simulink model "capitol6prob1"  (R2013a)
settings: Solver=ode45  StartTime=0.0  StopTime=200  RelTol=1e-3
undefined symbols (not defined in the file): des, gcbh
settings Model: Creator=user  LastModifiedBy=user

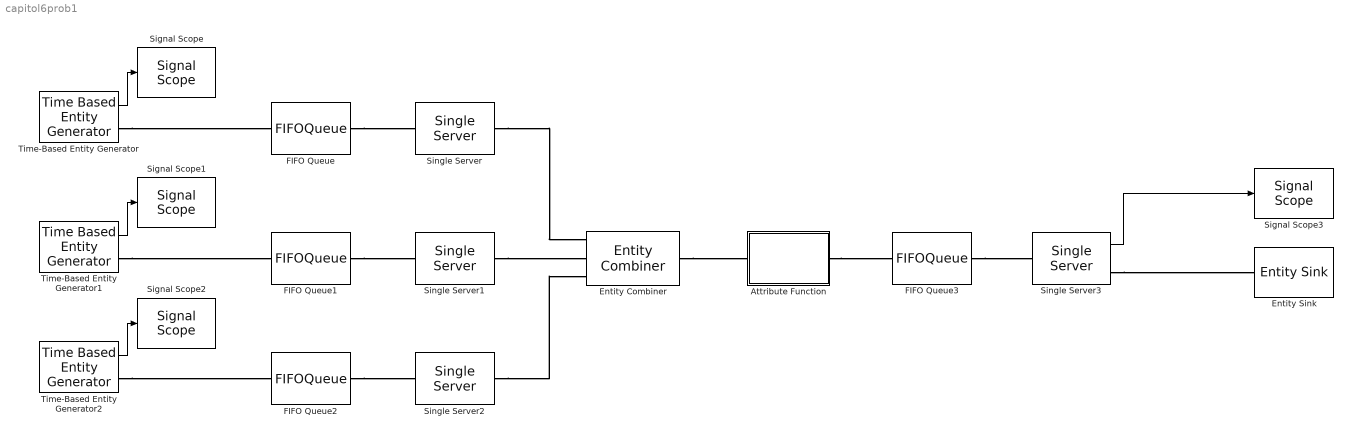
== system capitol6prob1 ==
  Attribute Function : Subsystem  LoadFcn=des.afb.attributefunction_support(gcb,'LoadFcn');  StartFcn=des.afb.attributefunction_support(gcb,'StartFcn');  mask(Attribute Function){OutputNamePrefix=out_}
      mask prompts: OutputNamePrefix "Prefix name"
      settings: CopyFcn=des.afb.attributefunction_support(gcb,'CopyFcn');  OpenFcn=des.afb.attributefunction_support(gcb,'OpenFcn');  ErrorFcn=des.afb.error_redirect
      mask Help: slhelp(gcbh)
      mask Display: image(des_iconLoad('attribFunction.jpg'),'center');
  Entity Combiner : EntityCombiner
  Entity Sink : EntitySink
  FIFO Queue{,1..3} (4 alike) : FIFOQueue
  Signal Scope{,1..3} (4 alike) : SignalScope  LoadFcn=des.scope.CallbackSupport('seLoadFcn',gcbh)  StartFcn=des.scope.CallbackSupport('seStartFcn',gcbh)  StopFcn=des.scope.CallbackSupport('seStopFcn',gcbh)
      settings: CopyFcn=des.scope.CallbackSupport('seCopyFcn',gcbh)  DeleteFcn=des.scope.CallbackSupport('seDeleteFcn',gcbh)  PreSaveFcn=des.scope.CallbackSupport('sePreSaveFcn',gcbh)  NameChangeFcn=des.scope.CallbackSupport('seNameChangeFcn',gcbh)  OpenFcn=des.scope.CallbackSupport('seOpenFcn',gcbh)
  Single Server : SingleServer  ServiceTime=0.6
  Single Server1 : SingleServer  ServiceTime=0.4
  Single Server2 : SingleServer  ServiceTime=0.4
  Single Server3 : SingleServer  ServiceTime=0.3  StatNumberDeparted=on
  Time-Based Entity Generator : TimeBasedEntityGenerator  Period=0.8  StatNumberDeparted=on
  Time-Based Entity Generator1 : TimeBasedEntityGenerator  Period=0.6  StatNumberDeparted=on
  Time-Based Entity Generator2 : TimeBasedEntityGenerator  Period=0.4  StatNumberDeparted=on
  wires:
  Time-Based Entity Generator/1 -> Signal Scope/1
  Time-Based Entity Generator1/1 -> Signal Scope1/1
  Time-Based Entity Generator2/1 -> Signal Scope2/1
  Single Server3/1 -> Signal Scope3/1
  connections:
  Time-Based Entity Generator2/RConn1 -- FIFO Queue2/LConn1
  Time-Based Entity Generator1/RConn1 -- FIFO Queue1/LConn1
  Time-Based Entity Generator/RConn1 -- FIFO Queue/LConn1
  FIFO Queue/RConn1 -- Single Server/LConn1
  FIFO Queue1/RConn1 -- Single Server1/LConn1
  FIFO Queue2/RConn1 -- Single Server2/LConn1
  Single Server/RConn1 -- Entity Combiner/LConn1
  Single Server1/RConn1 -- Entity Combiner/LConn2
  Single Server2/RConn1 -- Entity Combiner/LConn3
  FIFO Queue3/RConn1 -- Single Server3/LConn1
  Single Server3/RConn1 -- Entity Sink/LConn1
  Entity Combiner/RConn1 -- Attribute Function/LConn1
  Attribute Function/RConn1 -- FIFO Queue3/LConn1

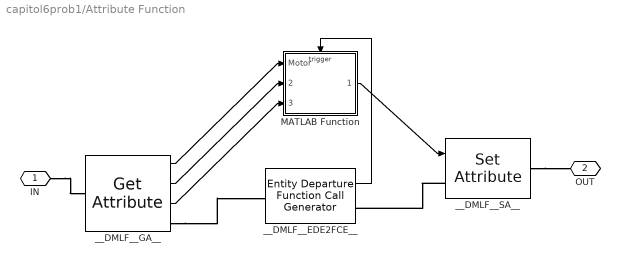
== system capitol6prob1/Attribute Function ==
  MATLAB Function : MATLAB Function  TreatAsAtomicUnit=on
  __DMLF__EDE2FCE__ : EntityDepartureFunctionCallGenerator  TimingFunctionCallF1=Before entity departure  IsInsideAFB=on
  __DMLF__GA__ : GetAttribute  AttributeName=Motor|Transmission|Chassis  AttributeMissing=Error|Error|Error  AttributeDefaultValue=1|1|1  AttributeTreatAsVector=1|1|1  AttributeSendTiming=Before entity departure|Before entity departure|Before entity departure  EvaluatedDefaultAttributeValue={ [];[];[]}  IsInsideAFB=on
      settings: OutputPortMap=o1,o2,o3
  __DMLF__SA__ : SetAttribute  AttributeName=Auto_Number  AttributeFrom=Signal port  EvaluatedAttributeValue={ []}  IsInsideAFB=on
  IN : PMIOPort  Port=1  Side=Left
  OUT : PMIOPort  Port=2  Side=Right
  wires:
  __DMLF__EDE2FCE__/1 -> MATLAB Function/Trigger
  __DMLF__GA__/1 -> MATLAB Function/1(Motor)
  __DMLF__GA__/2 -> MATLAB Function/2(Transmission)
  __DMLF__GA__/3 -> MATLAB Function/3(Chassis)
  MATLAB Function/1(out_Auto_Number) -> __DMLF__SA__/1
  connections:
  __DMLF__SA__/LConn1 -- __DMLF__EDE2FCE__/RConn1
  __DMLF__GA__/RConn1 -- __DMLF__EDE2FCE__/LConn1
  IN/RConn1 -- __DMLF__GA__/LConn1
  __DMLF__SA__/RConn1 -- OUT/RConn1

== matlab function capitol6prob1/Attribute Function/MATLAB Function ==
  data: Motor input; out_Auto_Number output; Transmission input; Chassis input
  events: trigger input FUNCTION_CALL_EVENT
function out_Auto_Number  = fcn(Motor, Transmission,Chassis)
%FCN    Access and modify attributes with MATLAB 
% 
% Input arguments must match the attribute names.
% Output arguments must be out_<AttributeName>,
% e.g., out_ServiceTime where ServiceTime is the attribute name.
% 
% The output attribute will be created if it is not present.
%

out_Auto_Number=Motor+10*Transmission+100*Chassis;
